simulink library "Fade"  (R2022b)
settings: Solver=VariableStepAuto  StartTime=0.0  StopTime=10.0  RelTol=1e-3
libraries: FadeBtc x1
settings Model: Creator=sk1042978  LastModifiedBy=kl13806
settings SolverCC: AlgebraicLoopSolver=TrustRegion
settings DebuggingCC: UnconnectedInputMsg=warning  UnconnectedOutputMsg=warning  UnconnectedLineMsg=warning  SFMachineParentedDataDiag=warning  ArithmeticOperatorsInVariantConditions=warning
settings ModelReferenceCC: EnableRefExpFcnMdlSchedulingChecks=on
settings SFSimCC: CustomCodeUndefinedFunction=UseInterfaceOnly
settings RTWCC: DLArmComputeVersion=19.05

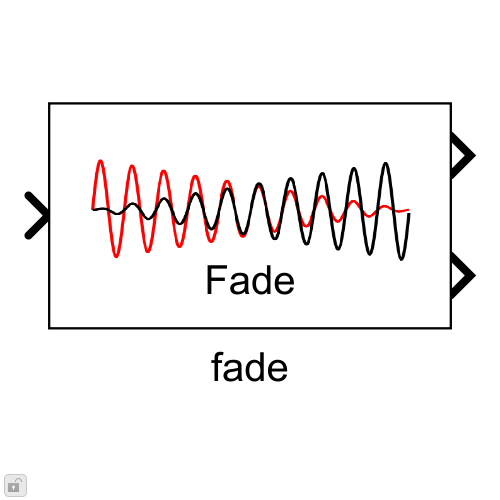
[thumbnail: Simulink's stored preview of the top-level diagram]
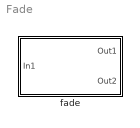
== system Fade ==
  fade : Subsystem  mask(Bose Fade){MaskFeatureName=Fade, MaskIndexOffset=128, MaskChanRampMap=[1,1,1,1,1,1,2,2,2,2,2,2], MaskSilentExtreme=on, MaskBoostDisable=off, MaskEnableGainPort=on, BankNumber=[], MaskPackageNumber=0}
      mask prompts: MaskFeatureName "Feature Name"; MaskIndexOffset "Index Offset"; MaskChanRampMap "Channel to ramper map"; MaskSilentExtreme "Enable silent extreme"; MaskBoostDisable "Disable Boost"; MaskEnableGainPort "Enable Output Gain Port"; BankNumber "Target memory bank number:"; MaskPackageNumber "Overlay package number"
      mask help: This block groups its input channels as 'Front' and 'Rear' and applies a fade forward or backward effect by using a combination of low pass and high pass filters.
      mask init:
      | blkh = gcbh;
      | % Copy discrete mask parameters into a classdef object
      | InnerLinkConfig = FadeConfig;
      | InnerLinkConfig.DefaultIndexOffset = MaskIndexOffset;
      | InnerLinkConfig.DefaultChanRampMap = MaskChanRampMap;
      | InnerLinkConfig.DefaultSilentExtreme = MaskSilentExtreme;
      | InnerLinkConfig.DefaultBoostDisable = MaskBoostDisable;
      | InnerLinkConfig.BankNumber = BankNumber;
      | 
      | EnableBlockPort(blkh,'Out2',MaskEnableGainPort);
      mask Help:
      | The Fade block includes runtime control support for adjusting the fade dynamically.
      | MASK PARAMETERS
      | - The Index offset determines the index which corresponds to the fade being in the center position (typically 128).
      | - Channels may to be assigned to either the Front ('1') or Rear ('2') groups. This field is set up as an array of channels with every channel assigned to atleast one valid group.
      | - 'Enable silent extreme' mutes the speakers of the group whose gains are being 'cut' when at extreme indices.
      | - 'Disable boost' determines whether a boost is required or not. If selected, the maximum boost will be '1' on the linear scale ('0' in dB), otherwise it is computed from the 'cut' gains (typically a maximum of 3 dB).
      | 
      | OUTPUTS
      | - audioOut
      | - fadeGains : 1x2 array [frontGain, rearGain]
      | 
      | RTC
      | Control messages can be sent through the RTC block. The block is configured to accept an index which determines the gains for each channel group, a ramp rate or time (the rate has precedence).
      | E.g., RTC_SIM_OBJ.AddREQ( 'FadeSet', 0.1, [0001, <fade_index>, <ramp_db_per_second>, <ramp_milliseconds>]);
      mask TypeOptions MaskFeatureName: InnerLink/FeatureName
      mask DialogControl ParameterText1 Prompt: The following operations are available to control the behavior of the block.
      mask DialogControl ParameterText3 Prompt: 'Index Scale' determines the total fade levels, while 'Index Offset' determines the index at which no fade is applied to the input audio. Input channels are to be mapped to either the 'Front' (1) or 'Rear' (2) channel groups. Enabling 'Silent extreme' mutes the speakers belonging to the opposite group, when the audio is faded completely forward or backward. 'Disable boost' sets the boost to 0 dB.
      mask Display:
      | image('Fade.png');
      | 
      | % retrieve the block's pixel size
      | pos = get(gcbh,'position');
      | bw = pos(3) - pos(1);
      | bh = pos(4) - pos(2);
      | 
      | % place feature name text
      | text(bw*0.5, 0, [MaskFeatureName '\n\n'], 'horizontalAlignment', 'center');

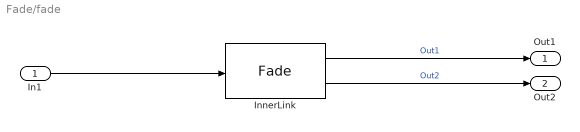
== system Fade/fade ==
  In1 : Inport
  InnerLink : FadeBtc/Fade  Config=InnerLinkConfig  FeatureName=Fade  EnableGainOut=on
      settings: SourceProductName=Bose Blocklib
  Out1 : Outport
  Out2 : Outport  Port=2
  wires:
  InnerLink/1 -> Out1/1  "Out1"
  InnerLink/2 -> Out2/1  "Out2"
  In1/1 -> InnerLink/1
